simulink model "cimulink2"  (R2021a)
settings: Solver=VariableStepAuto  StartTime=0.0  StopTime=10.0  RelTol=1e-3
settings Model: Creator=TUF GAMING  LastModifiedBy=TUF GAMING

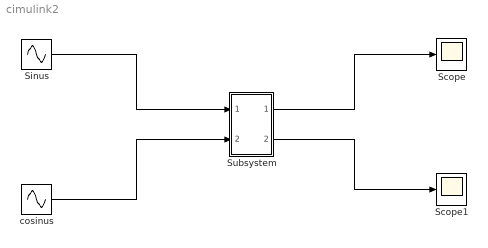
== system cimulink2 ==
  Scope : Scope
  Scope1 : Scope
  Sinus : Sin  SampleTime=0
  Subsystem : Subsystem
  cosinus : Sin  Phase=pi/2  SampleTime=0
  wires:
  Sinus/1 -> Subsystem/1(In1)
  cosinus/1 -> Subsystem/2(In2)
  Subsystem/1(Out1) -> Scope/1
  Subsystem/2(Out2) -> Scope1/1

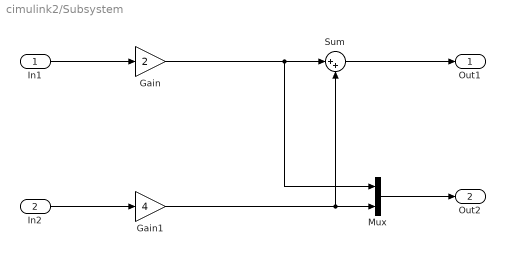
== system cimulink2/Subsystem ==
  In1 : Inport
  In2 : Inport  Port=2
  Gain : Gain  Gain=2
  Gain1 : Gain  Gain=4
  Mux : Mux  Inputs=2
  Sum : Sum  Inputs=|++
  Out1 : Outport
  Out2 : Outport  Port=2
  wires:
  In1/1 -> Gain/1
  Gain1/1 -> Mux/2, Sum/2
  Gain/1 -> Mux/1, Sum/1
  In2/1 -> Gain1/1
  Mux/1 -> Out2/1
  Sum/1 -> Out1/1
